simulink model "test"  (R2024b)
settings: Solver=ode1be  StartTime=0.0  StopTime=t_sim  FixedStep=T_sw/(2^PWM_resolution)  RelTol=1e-3
values from neighbouring files (symbols this model uses):
  PWM_resolution = 7    [init_digital_controller.m]
  t_sim = T_sw * 1000    (= 0.01)    [init.m]    (also in init_general.m = 0.005)
  T_sw = 1 / f_sw    (= 1e-05)    [init.m]    (also in init_general.m = 5e-06)
  v_PWM_max = 1    [init_digital_controller.m]
undefined symbols (not defined in the file or in its folder): comp_den_d, comp_num_d, dspblkCoreblockFVToolHelper, gcbh, N, v_ref
libraries: simulink x3
settings Model: Creator=hgholab  LastModifiedBy=hgholab

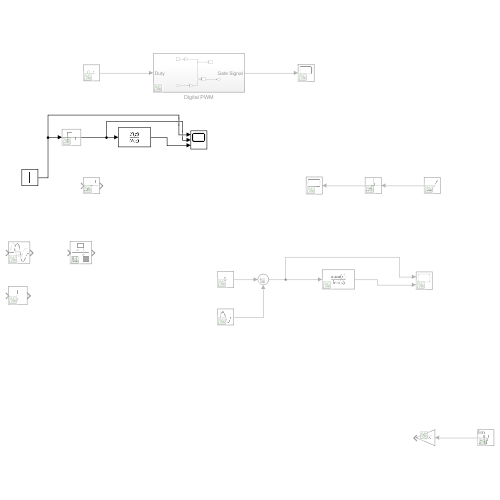
[thumbnail: Simulink's stored preview of the top-level diagram]
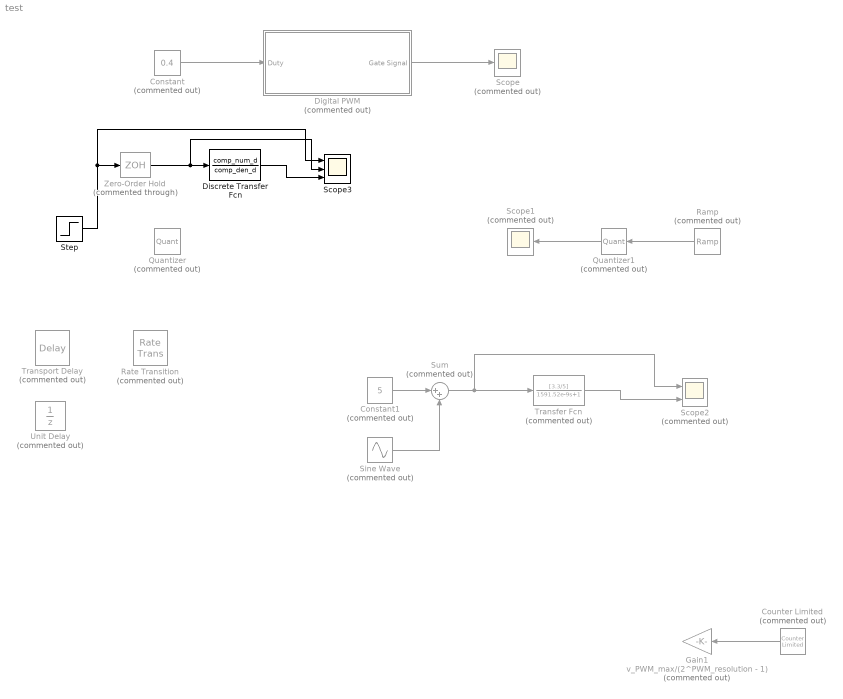
== system test ==
  Constant : Constant  Commented=on  Value=0.4
  Constant1 : Constant  Commented=on  Value=5
  Counter Limited : simulink/Sources/Counter Limited  Commented=on  uplimit=2^PWM_resolution - 1  tsamp=T_sw/N
  Digital PWM : Subsystem  Commented=on
  Discrete Transfer Fcn : DiscreteTransferFcn  LoadFcn=dspblkCoreblockFVToolHelper(gcbh,'load');  Numerator=comp_num_d  Denominator=comp_den_d
      settings: CopyFcn=dspblkCoreblockFVToolHelper(gcbh,'copy');  DeleteFcn=dspblkCoreblockFVToolHelper(gcbh,'close');  ModelCloseFcn=dspblkCoreblockFVToolHelper(gcbh,'close');  PreSaveFcn=dspblkCoreblockFVToolHelper(gcbh,'presave');  PostSaveFcn=dspblkCoreblockFVToolHelper(gcbh,'postsave');  CloseFcn=dspblkCoreblockFVToolHelper(gcbh,'close');
  Gain1 : Gain  Commented=on  Gain=v_PWM_max/(2^PWM_resolution - 1)
  Quantizer : Quantizer  Commented=on  QuantizationInterval=v_ref/N
  Quantizer1 : Quantizer  Commented=on  QuantizationInterval=v_ref/N
  Ramp : simulink/Sources/Ramp  Commented=on  slope=2/t_sim  start=0  InitialOutput=-1
  Rate Transition : RateTransition  Commented=on
  Scope : Scope  Commented=on
  Scope1 : Scope  Commented=on
  Scope2 : Scope  Commented=on  NumInputPorts=2
  Scope3 : Scope  NumInputPorts=3
  Sine Wave : Sin  Commented=on  Amplitude=0.040  Frequency=200000*2*pi  SampleTime=0
  Step : Step  Time=0  SampleTime=0
  Sum : Sum  Commented=on  Inputs=|++
  Transfer Fcn : TransferFcn  Commented=on  Numerator=[3.3/5]  Denominator=[1591.52e-9 1]
  Transport Delay : TransportDelay  Commented=on
  Unit Delay : UnitDelay  Commented=on  SampleTime=-1  HasFrameUpgradeWarning=on
  Zero-Order Hold : ZeroOrderHold  Commented=through  SampleTime=-1
  wires:
  Constant/1 -> Digital PWM/1(Duty)
  Digital PWM/1(Gate Signal) -> Scope/1
  Ramp/1 -> Quantizer1/1
  Quantizer1/1 -> Scope1/1
  Transfer Fcn/1 -> Scope2/2
  Constant1/1 -> Sum/1
  Sine Wave/1 -> Sum/2
  Sum/1 -> Scope2/1, Transfer Fcn/1
  Counter Limited/1 -> Gain1/1
  Zero-Order Hold/1 -> Scope3/2, Discrete Transfer Fcn/1
  Step/1 -> Scope3/1, Zero-Order Hold/1
  Discrete Transfer Fcn/1 -> Scope3/3

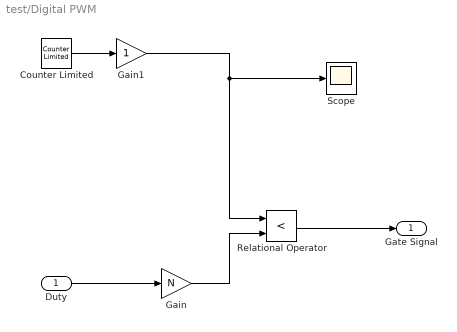
== system test/Digital PWM ==
  Duty : Inport
  Counter Limited : simulink/Sources/Counter Limited  uplimit=N - 1  tsamp=T_sw/N
  Gain : Gain  Gain=N
  Gain1 : Gain
  Relational Operator : RelationalOperator  Operator=<  OutDataTypeStr=boolean  RndMeth=Simplest  InputSameDT=off
  Scope : Scope
  Gate Signal : Outport
  wires:
  Duty/1 -> Gain/1
  Counter Limited/1 -> Gain1/1
  Gain/1 -> Relational Operator/2
  Relational Operator/1 -> Gate Signal/1
  Gain1/1 -> Relational Operator/1, Scope/1
